simulink model "Baxter_brake_flex_sim"  (R2017b)
settings: Solver=ode8  StartTime=0.0  StopTime=T  FixedStep=0.0001  RelTol=5e-2  EnableMultiTasking=on
values from neighbouring files (symbols this model uses):
  A0 = zeros(6,1)    [friction_braking_analysis.m]    (also in friction_braking_analysis_flex.m)
  Ic = [(0.5*m*(3*r^2 + ht^2)) 0 0; 0 (0.5*m*(3*r^2 + ht^2)) 0;      0 0 0.5*m*r^2]    [friction_braking_analysis.m]    (also in friction_braking_analysis_flex.m; trap_traj_gen_check.m)
  Mc_inv = inv(Mc)    [friction_braking_analysis.m]    (also in friction_braking_analysis_flex.m; trap_traj_gen_check.m)
  N = length(lambda)-1    [trap_traj_gen_check.m]
  qdotIC = qIC    [friction_braking_analysis.m]    (also in friction_braking_analysis_flex.m)
  qIC = zeros(7,1)    [friction_braking_analysis.m]    (also in friction_braking_analysis_flex.m)
  qmdotIC = KN_inv*(Mdot*qddotIC + MassInertia*qjerkIC + Cdot*qdotIC +      C*qddotIC + Fdot + Ks*Ns*Ns*qdotIC + Jdot'*f + J'*fdot)    [friction_braking_analysis_flex.m]
  qmIC = KN_inv*(MassInertia*qddotIC + Cq + F + Ks*Ns*Ns*qIC +J'*f)    [friction_braking_analysis_flex.m]
  ric_tip = PTs    [friction_braking_analysis.m]    (also in friction_braking_analysis_flex.m; trap_traj_gen_check.m)
  Tb = 10*ones(7,1)    [friction_braking_analysis.m]    (also in friction_braking_analysis_flex.m)
  Tc = [1;1;1;1;0.5;0.5;0.5]    [friction_braking_analysis.m]    (also in friction_braking_analysis_flex.m)
  V0 = zeros(6,1)    [friction_braking_analysis.m]    (also in friction_braking_analysis_flex.m)
undefined symbols (not defined in the file or in its folder): qdotlimit, robot_const
libraries: simulink x1
settings Model: Creator=davidcarabis  LastModifiedBy=davidcarabis
settings SolverCC: MaxConsecutiveMinStep=10  ZeroCrossControl=EnableAll
settings DataIOCC: LimitDataPoints=on  SaveFormat=Array
settings OptimizationCC: LifeSpan=inf
settings DebuggingCC: ReadBeforeWriteMsg=DisableAll  WriteAfterWriteMsg=DisableAll  WriteAfterReadMsg=DisableAll  MultiTaskDSMMsg=none  SFUnexpectedBacktrackingDiag=warning  SFNoUnconditionalDefaultTransitionDiag=warning  SFExecutionAtInitializationDiag=none
settings HardwareCC: ProdBitPerPointer=32  ProdBitPerSizeT=32  ProdBitPerPtrDiffT=32  ProdLargestAtomicFloat=None  ProdIntDivRoundTo=Undefined  ProdEndianess=Unspecified  ProdWordSize=32  ProdHWDeviceType=32-bit Generic
settings ModelReferenceCC: UpdateModelReferenceTargets=IfOutOfDate  PropagateSignalLabelsOutOfModel=off
settings SFSimCC: SFSimEcho=off
settings CodeAppCC: StateflowObjectComments=on
settings GRTTargetCC: TargetLangStandard=C89/C90 (ANSI)  GeneratePreprocessorConditionals=Disable all
settings ConfigComp: CovMetricSettings=dw  CovHtmlReporting=on  CovSaveCumulativeToWorkspaceVar=on  CovSaveSingleToWorkspaceVar=on  CovExternalEMLEnable=off

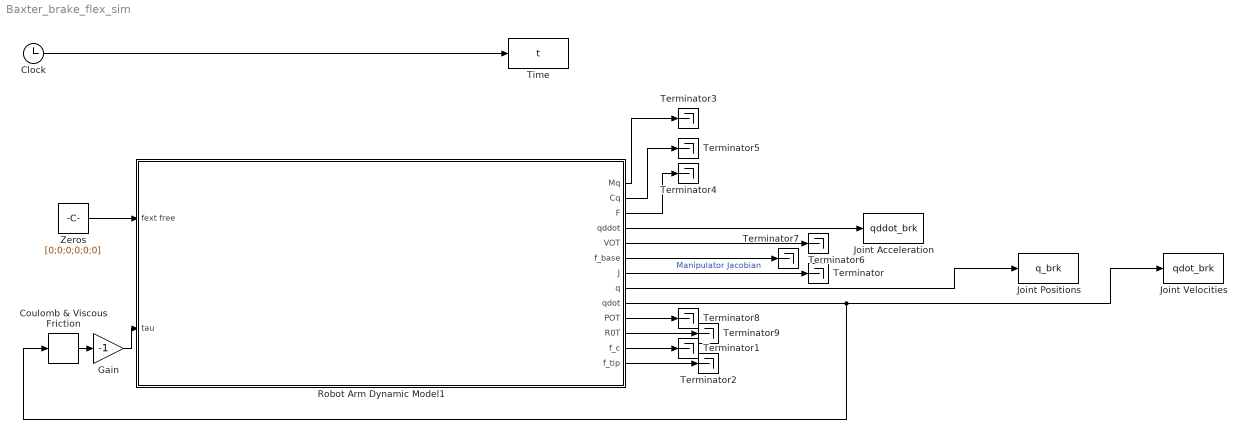
== system Baxter_brake_flex_sim ==
  Clock : Clock
  Coulomb & Viscous Friction : simulink/Discontinuities/Coulomb & Viscous Friction  offset=[Tc(1) Tc(2) Tc(3) Tc(4) Tc(5) Tc(6) Tc(7)]  gain=[Tb(1) Tb(2) Tb(3) Tb(4) Tb(5) Tb(6) Tb(7)]
      settings: SourceProductName=Simulink
  Gain : Gain  Gain=-1
  Joint Acceleration : ToWorkspace  VariableName=qddot_brk  SampleTime=-1
  Joint Positions : ToWorkspace  VariableName=q_brk  SampleTime=-1
  Joint Velocities : ToWorkspace  VariableName=qdot_brk  SampleTime=-1
  Robot Arm Dynamic Model1 : Subsystem
  Terminator{,1..9} (10 alike) : Terminator
  Time : ToWorkspace  VariableName=t  SampleTime=-1
  Zeros : Constant  Value=[0;0;0;0;0;0]
  wires:
  Clock/1 -> Time/1
  Robot Arm Dynamic Model1/9(qdot) -> Coulomb & Viscous Friction/1, Joint Velocities/1
  Robot Arm Dynamic Model1/8(q) -> Joint Positions/1
  Zeros/1 -> Robot Arm Dynamic Model1/1(fext free)
  Robot Arm Dynamic Model1/4(qddot) -> Joint Acceleration/1
  Robot Arm Dynamic Model1/7(J) -> Terminator/1  "Manipulator Jacobian"
  Robot Arm Dynamic Model1/12(f_c) -> Terminator1/1
  Robot Arm Dynamic Model1/13(f_tip) -> Terminator2/1
  Robot Arm Dynamic Model1/1(Mq) -> Terminator3/1
  Robot Arm Dynamic Model1/2(Cq) -> Terminator5/1
  Robot Arm Dynamic Model1/3(F) -> Terminator4/1
  Robot Arm Dynamic Model1/5(VOT) -> Terminator6/1
  Robot Arm Dynamic Model1/6(f_base) -> Terminator7/1
  Robot Arm Dynamic Model1/10(POT) -> Terminator8/1
  Robot Arm Dynamic Model1/11(R0T) -> Terminator9/1
  Coulomb & Viscous Friction/1 -> Gain/1
  Gain/1 -> Robot Arm Dynamic Model1/2(tau)

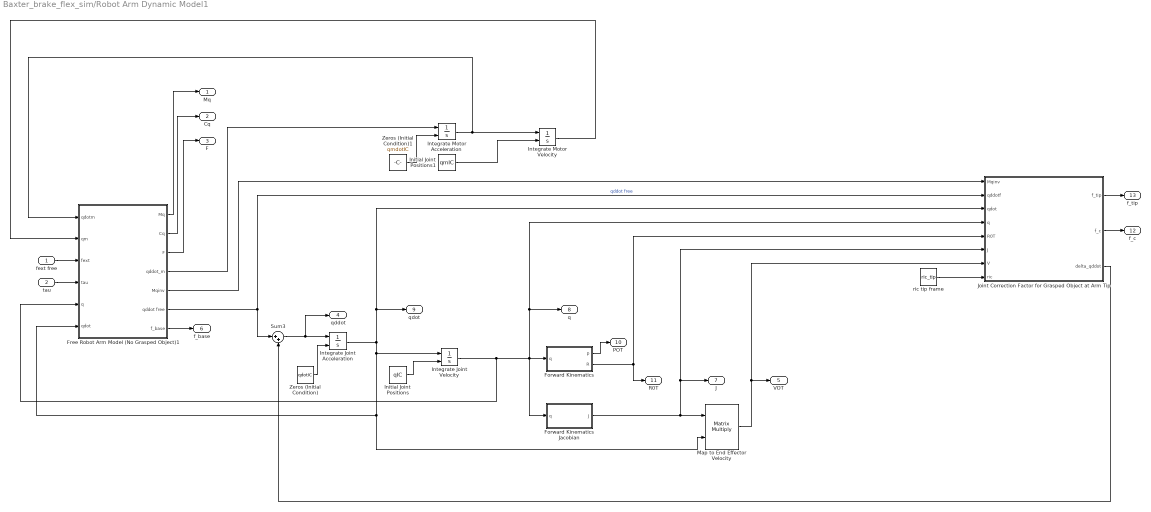
== system Baxter_brake_flex_sim/Robot Arm Dynamic Model1 ==
  fext free : Inport
  tau : Inport  Port=2
  Forward Kinematics : Subsystem  mask{H=robot_const.kin.H, P=robot_const.kin.P}
      mask prompts: H "Actuator Axes"; P "Actuator Displacements"
  Forward Kinematics Jacobian : Subsystem  mask{H=robot_const.kin.H, P=robot_const.kin.P}
      mask prompts: H "Actuator Axes"; P "Actuator Displacements"
  Free Robot Arm Model (No Grasped Object)1 : Subsystem
  Initial Joint Positions : Constant  Value=qIC
  Initial Joint Positions1 : Constant  Value=qmIC
  Integrate Joint Acceleration : Integrator  InitialConditionSource=external  InitialCondition=[0;0;0;0;0;0;0]
  Integrate Joint Velocity : Integrator  InitialConditionSource=external  InitialCondition=[0;0;0;0;0;0;0]
  Integrate Motor Acceleration : Integrator  InitialConditionSource=external  InitialCondition=[0;0;0;0;0;0;0]  UpperSaturationLimit=qdotlimit(:,2).*N  LowerSaturationLimit=qdotlimit(:,1).*N
  Integrate Motor Velocity : Integrator  InitialConditionSource=external  InitialCondition=[0;0;0;0;0;0;0]
  Joint Correction Factor for Grasped Object at Arm Tip : Subsystem  mask{Ic=Ic, Mcinv=Mc_inv}
  Map to End Effector Velocity : Product  Multiplication=Matrix(*)
  Sum3 : Sum  Inputs=|++
  Zeros (Initial Condition) : Constant  Value=qdotIC
  Zeros (Initial Condition)1 : Constant  Value=qmdotIC
  ric tip frame : Constant  Value=ric_tip
  Mq : Outport
  Cq : Outport  Port=2
  F : Outport  Port=3
  qddot : Outport  Port=4
  VOT : Outport  Port=5
  f_base : Outport  Port=6
  J : Outport  Port=7
  q : Outport  Port=8
  qdot : Outport  Port=9
  POT : Outport  Port=10
  R0T : Outport  Port=11
  f_c : Outport  Port=12
  f_tip : Outport  Port=13
  wires:
  Forward Kinematics/1(p) -> POT/1
  Integrate Joint Velocity/1 -> Free Robot Arm Model (No Grasped Object)1/5("q "), Forward Kinematics Jacobian/1(q), Forward Kinematics/1(q), Joint Correction Factor for Grasped Object at Arm Tip/4(q), q/1
  Zeros (Initial Condition)/1 -> Integrate Joint Acceleration/2
  fext free/1 -> Free Robot Arm Model (No Grasped Object)1/3(fext)
  Initial Joint Positions/1 -> Integrate Joint Velocity/2
  Forward Kinematics Jacobian/1(J) -> J/1, Joint Correction Factor for Grasped Object at Arm Tip/6(J), Map to End Effector Velocity/1
  Map to End Effector Velocity/1 -> Joint Correction Factor for Grasped Object at Arm Tip/7(V), VOT/1
  Integrate Joint Acceleration/1 -> Free Robot Arm Model (No Grasped Object)1/6(qdot), Map to End Effector Velocity/2, Integrate Joint Velocity/1, Joint Correction Factor for Grasped Object at Arm Tip/3(qdot), qdot/1
  tau/1 -> Free Robot Arm Model (No Grasped Object)1/4(tau)
  Forward Kinematics/2(R) -> Joint Correction Factor for Grasped Object at Arm Tip/5(R0T), R0T/1
  Free Robot Arm Model (No Grasped Object)1/7(f_base) -> f_base/1
  Free Robot Arm Model (No Grasped Object)1/5(Mqinv) -> Joint Correction Factor for Grasped Object at Arm Tip/1(Mqinv)
  Free Robot Arm Model (No Grasped Object)1/1(Mq) -> Mq/1
  Free Robot Arm Model (No Grasped Object)1/2(Cq) -> Cq/1
  Free Robot Arm Model (No Grasped Object)1/3(F) -> F/1
  Free Robot Arm Model (No Grasped Object)1/6(qddot free) -> Joint Correction Factor for Grasped Object at Arm Tip/2(qddotf), Sum3/1  "qddot free"
  Sum3/1 -> qddot/1, Integrate Joint Acceleration/1
  Joint Correction Factor for Grasped Object at Arm Tip/3(delta_qddot) -> Sum3/2
  Joint Correction Factor for Grasped Object at Arm Tip/2(f_c) -> f_c/1
  Joint Correction Factor for Grasped Object at Arm Tip/1(f_tip) -> f_tip/1
  ric tip frame/1 -> Joint Correction Factor for Grasped Object at Arm Tip/8(ric)
  Integrate Motor Acceleration/1 -> Free Robot Arm Model (No Grasped Object)1/1(qdotm), Integrate Motor Velocity/1
  Integrate Motor Velocity/1 -> Free Robot Arm Model (No Grasped Object)1/2(qm)
  Initial Joint Positions1/1 -> Integrate Motor Velocity/2
  Free Robot Arm Model (No Grasped Object)1/4(qddot_m) -> Integrate Motor Acceleration/1
  Zeros (Initial Condition)1/1 -> Integrate Motor Acceleration/2

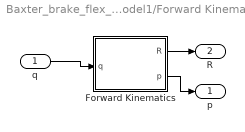
== system Baxter_brake_flex_sim/Robot Arm Dynamic Model1/Forward Kinematics ==
  q : Inport
  Forward Kinematics : MATLAB Function  TreatAsAtomicUnit=on
  p : Outport
  R : Outport  Port=2
  wires:
  q/1 -> Forward Kinematics/1(q)
  Forward Kinematics/2(p) -> p/1
  Forward Kinematics/1(R) -> R/1

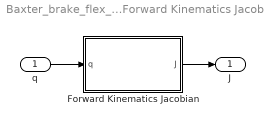
== system Baxter_brake_flex_sim/Robot Arm Dynamic Model1/Forward Kinematics Jacobian ==
  q : Inport
  Forward Kinematics Jacobian : MATLAB Function  TreatAsAtomicUnit=on
  J : Outport
  wires:
  q/1 -> Forward Kinematics Jacobian/1(q)
  Forward Kinematics Jacobian/1(J) -> J/1

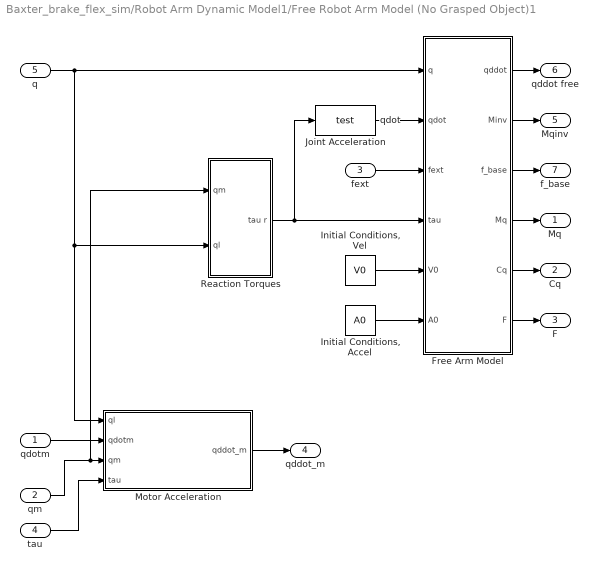
== system Baxter_brake_flex_sim/Robot Arm Dynamic Model1/Free Robot Arm Model (No Grasped Object)1 ==
  qdotm : Inport
  qm : Inport  Port=2
  fext : Inport  Port=3
  tau : Inport  Port=4
  "q " : Inport  Port=5
  qdot : Inport  Port=6
  Free Arm Model : Subsystem  mask{h=robot_const.kin.H, p=robot_const.kin.P, m=robot_const.mprops.m, c=robot_const.mprops.c, I=robot_const.mprops.I, Im=robot_const.mprops.Im, N=robot_const.mprops.N}
      mask prompts: h "Actuator Axes"; p "Actuator Displacements"; m "Link Masses"; c "Link COM"; I "Link Inertia"; N "Gear Ratio"
  "Initial Conditions, Accel" : Constant  Value=A0
  "Initial Conditions, Vel" : Constant  Value=V0
  Joint Acceleration : ToWorkspace  VariableName=test  SampleTime=-1
  Motor Acceleration : Subsystem  mask{Im=robot_const.mprops.Im, N=robot_const.mprops.N, K=robot_const.mprops.K}
      mask prompts: Im "Motor Inertias"; N "Gear Ratios"; K "Joint Stiffnesses"
  Reaction Torques : Subsystem  mask{N=robot_const.mprops.N, K=robot_const.mprops.K}
      mask prompts: N "Gear Ratios"; K "Joint Stiffnesses"
  Mq : Outport
  Cq : Outport  Port=2
  F : Outport  Port=3
  qddot_m : Outport  Port=4
  Mqinv : Outport  Port=5
  qddot free : Outport  Port=6
  f_base : Outport  Port=7
  wires:
  "q "/1 -> Reaction Torques/2(ql), Motor Acceleration/1(ql), Free Arm Model/1(q)
  fext/1 -> Free Arm Model/3(fext)
  qdot/1 -> Free Arm Model/2(qdot)
  "Initial Conditions, Vel"/1 -> Free Arm Model/5(V0)
  "Initial Conditions, Accel"/1 -> Free Arm Model/6(A0)
  Free Arm Model/1(qddot) -> qddot free/1
  Free Arm Model/2(Minv) -> Mqinv/1
  Free Arm Model/3(f_base) -> f_base/1
  Free Arm Model/4(Mq) -> Mq/1
  Free Arm Model/5(Cq) -> Cq/1
  Free Arm Model/6(F) -> F/1
  tau/1 -> Motor Acceleration/4(tau)
  Motor Acceleration/1(qddot_m) -> qddot_m/1
  qm/1 -> Reaction Torques/1(qm), Motor Acceleration/3(qm)
  qdotm/1 -> Motor Acceleration/2(qdotm)
  Reaction Torques/1(tau r) -> Joint Acceleration/1, Free Arm Model/4(tau)

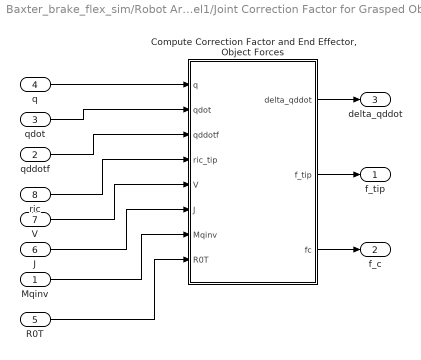
== system Baxter_brake_flex_sim/Robot Arm Dynamic Model1/Joint Correction Factor for Grasped Object at Arm Tip ==
  Mqinv : Inport
  qddotf : Inport  Port=2
  qdot : Inport  Port=3
  q : Inport  Port=4
  R0T : Inport  Port=5
  J : Inport  Port=6
  V : Inport  Port=7
  ric : Inport  Port=8
  "Compute Correction Factor and End Effector, Object Forces" : MATLAB Function  TreatAsAtomicUnit=on
  f_tip : Outport
  f_c : Outport  Port=2
  delta_qddot : Outport  Port=3
  wires:
  q/1 -> "Compute Correction Factor and End Effector, Object Forces"/1(q)
  "Compute Correction Factor and End Effector, Object Forces"/1(delta_qddot) -> delta_qddot/1
  J/1 -> "Compute Correction Factor and End Effector, Object Forces"/6(J)
  qddotf/1 -> "Compute Correction Factor and End Effector, Object Forces"/3(qddotf)
  ric/1 -> "Compute Correction Factor and End Effector, Object Forces"/4(ric_tip)
  qdot/1 -> "Compute Correction Factor and End Effector, Object Forces"/2(qdot)
  V/1 -> "Compute Correction Factor and End Effector, Object Forces"/5(V)
  Mqinv/1 -> "Compute Correction Factor and End Effector, Object Forces"/7(Mqinv)
  R0T/1 -> "Compute Correction Factor and End Effector, Object Forces"/8(R0T)
  "Compute Correction Factor and End Effector, Object Forces"/2(f_tip) -> f_tip/1
  "Compute Correction Factor and End Effector, Object Forces"/3(fc) -> f_c/1

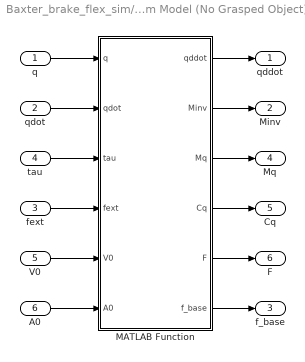
== system Baxter_brake_flex_sim/Robot Arm Dynamic Model1/Free Robot Arm Model (No Grasped Object)1/Free Arm Model ==
  q : Inport
  qdot : Inport  Port=2
  fext : Inport  Port=3
  tau : Inport  Port=4
  V0 : Inport  Port=5
  A0 : Inport  Port=6
  MATLAB Function : MATLAB Function  TreatAsAtomicUnit=on
  qddot : Outport
  Minv : Outport  Port=2
  f_base : Outport  Port=3
  Mq : Outport  Port=4
  Cq : Outport  Port=5
  F : Outport  Port=6
  wires:
  MATLAB Function/1(qddot) -> qddot/1
  q/1 -> MATLAB Function/1(q)
  fext/1 -> MATLAB Function/4(fext)
  tau/1 -> MATLAB Function/3(tau)
  V0/1 -> MATLAB Function/5(V0)
  qdot/1 -> MATLAB Function/2(qdot)
  A0/1 -> MATLAB Function/6(A0)
  MATLAB Function/2(Minv) -> Minv/1
  MATLAB Function/6(f_base) -> f_base/1
  MATLAB Function/3(Mq) -> Mq/1
  MATLAB Function/4(Cq) -> Cq/1
  MATLAB Function/5(F) -> F/1

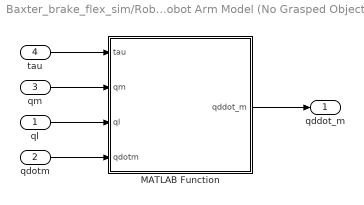
== system Baxter_brake_flex_sim/Robot Arm Dynamic Model1/Free Robot Arm Model (No Grasped Object)1/Motor Acceleration ==
  ql : Inport
  qdotm : Inport  Port=2
  qm : Inport  Port=3
  tau : Inport  Port=4
  MATLAB Function : MATLAB Function  TreatAsAtomicUnit=on
  qddot_m : Outport
  wires:
  ql/1 -> MATLAB Function/3(ql)
  tau/1 -> MATLAB Function/1(tau)
  qm/1 -> MATLAB Function/2(qm)
  MATLAB Function/1(qddot_m) -> qddot_m/1
  qdotm/1 -> MATLAB Function/4(qdotm)

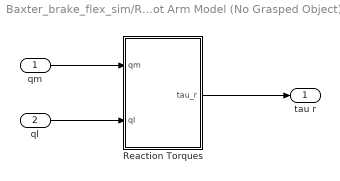
== system Baxter_brake_flex_sim/Robot Arm Dynamic Model1/Free Robot Arm Model (No Grasped Object)1/Reaction Torques ==
  qm : Inport
  ql : Inport  Port=2
  Reaction Torques : MATLAB Function  TreatAsAtomicUnit=on
  tau r : Outport
  wires:
  qm/1 -> Reaction Torques/1(qm)
  ql/1 -> Reaction Torques/2(ql)
  Reaction Torques/1(tau_r) -> tau r/1

== matlab function Baxter_brake_flex_sim/Robot Arm Dynamic Model1/Forward Kinematics/Forward Kinematics ==
  data: R output; q input; p output; H parameter; P parameter
function [R, p] = FwdKin(q,H,P)
%#codegen

% Generates robot pose from forward Kinematics
% Inputs:
% q: vector of joint positions
% H: matrix of joint unit vectors
% P: matrix of joint offsets
%
% Outputs:
% R: orientation (rotation matrix)
% P: position
%
%%%%%%%%%%%%%%%%%%%%%%%%%%%%%%%%%%%%%%%%%%%%%%%%%%%%%%%%%%%%%%%%%%%%%%%%%%%

    n = size(H,2);
    
    p = P(:,1);
    R = eye(3);
        
    for i=1:n
        R = R*rot(H(:,i),q(i));
        p = p + R*P(:,i+1);
    end
    
end

== matlab function Baxter_brake_flex_sim/Robot Arm Dynamic Model1/Forward Kinematics Jacobian/Forward Kinematics Jacobian ==
  data: J output; q input; H parameter; P parameter
function J = robotjacobian(q,H,P)
%#codegen

% Generates manipulator Jacobian using forward kinematics.
%
% Inputs: 
% q: vector of joint positions
% H: matrix of joint unit vectors
% P: matrix of joint offsets
%
% Outputs:
% J: manipulator Jacobian

%%%%%%%%%%%%%%%%%%%%%%%%%%%%%%%%%%%%%%%%%%%%%%%%%%%%%%%%%%%%%%%%%%%%%%%%%%%
    n = size(H,2);
    
    p = P(:,1);
    R = eye(3);
    
    hi = zeros(3,n);
    pOi = P;
        
    for i=1:n
        R = R*rot(H(:,i),q(i));
        p = p + R*P(:,i+1);
        pOi(:,i+1) = p;
        hi(:,i) = R*H(:,i);
    end
    
    pOT = pOi(:,end);
    J = zeros(6,n);
    
    for i=1:n
        J(:,i) = [hi(:,i); hat(hi(:,i))*(pOT - pOi(:,i))];
    end
    
end

== matlab function Baxter_brake_flex_sim/Robot Arm Dynamic Model1/Free Robot Arm Model (No Grasped Object)1/Free Arm Model/MATLAB Function ==
  data: q input; qddot output; qdot input; tau input; fext input; h parameter; p parameter; V0 input; A0 input; I parameter; m parameter; c parameter; Minv output; Mq output; Cq output; F output; f_base output; Im parameter; N parameter
function [qddot,Minv,Mq,Cq,F,f_base] = fcn(q,qdot,tau,fext,h,p,V0,A0,I,m,c,Im,N)
%#codegen

% This code computes the free dynamics of the Baxter arm using the N-E
% formulation. The free dynamics assumption is that there is no load at the
% tip of the manipulator arm.
%
% The N-E formulation is as follows for the ith joint:
% f_i = P_i*A_i + B_i
% First, a forward sweep computes spatial velocity of each point. 
% Next, a reverse sweep computes P, B for each joint.
% Finally, a forward sweep computes spatial acceleration, force, and joint
% acceleration.
%
% Inputs: 
% q: joint positions
% qdot: joint velocities
% tau: applied joint torques from motor/controller
% fext: external spatial force (should be set to zero)
% h: joint vectors of rotation
% p: joint offsets
% V0: spatial velocity initial condition
% A0: spatial acceleration initial condition
% I: equivalent manipulator link inertia matrices (accounts for motor 
%       inertia), at center of mass, represented in the ith frame for the
%       ith link
% m: manpulator link masses
% c: vectors from ith frame to ith link center of mass, represented in ith
%       frame
%
% Outputs:
% qddot: joint accelerations for free manipulator arm model
% Minv: inverse of the manipulator arm mass inertia matrix - this is needed
%       for the joint acceleration correction due to load at the tip
% f_base: spatial force at arm base

%%%%%%%%%%%%%%%%%%%%%%%%%%%%%%%%%%%%%%%%%%%%%%%%%%%%%%%%%%%%%%%%%%%%%%%%%%%

% Generate H, PHI block matrices

H1 = [h(:,1); 0;0;0]; H2 = [h(:,2); 0;0;0]; H3 = [h(:,3); 0;0;0]; 
H4 = [h(:,4); 0;0;0]; H5 = [h(:,5); 0;0;0]; H6 = [h(:,6); 0;0;0]; 
H7 = [h(:,7); 0;0;0];

H = [H1 zeros(6,6); zeros(6,1) H2 zeros(6,5); zeros(6,2) H3 zeros(6,4); ...
    zeros(6,3) H4 zeros(6,3); zeros(6,4) H5 zeros(6,2); zeros(6,5) H6 ...
    zeros(6,1); zeros(6,6) H7];

PHI = phi_gen(q,h,p);

N = diag(N);

%% Forward Sweep - Compute V,a,b, M
% V is spatial velocity of each joint.
% a,b are terms that will be used in later computations.
% Compute mass-inertia matrices for each link (M)

V = zeros(6,7);
Vtemp = V0;
Vprev = V0;
a = zeros(6,7);
b = zeros(6,7);
M = zeros(6,6,7);
M_motors = zeros(6,6,7);

for k = 1:7
   PHI_TEMP = PHI((6*(k) - 5):(6*(k)),(6*(k) - 5):(6*(k)));
   Htemp = H((6*(k) - 5):(6*(k)),k);
   Vtemp = PHI_TEMP*Vtemp + Htemp*qdot(k);
   V(:,k) = Vtemp;
   
   R = rot(H(:,k),q(k));
   
   a(:,k) = [crossmat(R'*Vprev(1:3))*(Vtemp(1:3));...
        R'*crossmat(Vprev(1:3))*(crossmat(Vprev(1:3))*p(:,k))];
   Vprev = Vtemp;
   
   b(:,k) = [crossmat(Vtemp(1:3))*I(:,:,k)*Vtemp(1:3); ...
        m(k)*crossmat(Vtemp(1:3))*crossmat(Vtemp(1:3))*c(:,k)];
    
    
    M(:,:,k) =  [I(:,:,k) m(k)*crossmat(c(:,k)); ...
        -m(k)*crossmat(c(:,k)) m(k)*eye(3,3)];
    M_motors(:,:,k) = [(I(:,:,k)+Im(k)*N(k,k)^2*h(:,k)*h(:,k)') m(k)*crossmat(c(:,k)); ...
        -m(k)*crossmat(c(:,k)) m(k)*eye(3,3)];
end

%% Backward Sweep for P, B
% Find P, B for each joint using reverse sweep.

F = -friction_adjust_Baxter(zeros(7,1),N*qdot);

P = zeros(6,6,7);
B = zeros(6,6,7);

% Handle Boundary Condition First
PHIT7 = [eye(3,3) zeros(3,3); -eye(3,3)*crossmat(p(:,8)) eye(3,3)];
P(:,:,7) = M(:,:,7);
B(:,7) = PHIT7'*fext + b(:,7);

% reverse sweep to compute other terms
for k = 6:-1:1
    PHI_TEMP = PHI((6*(k) +1):(6*(k)+6),(6*(k) +1):(6*(k) + 6));
    Htemp = H((6*(k) +1):(6*(k))+6,k+1);
    P(:,:,k) = M(:,:,k) + PHI_TEMP'*P(:,:,k+1)*PHI_TEMP - ...
        (PHI_TEMP'*P(:,:,k+1)*Htemp*Htemp'*P(:,:,k+1)*PHI_TEMP)/...
        (Htemp'*P(:,:,k+1)*Htemp);
    
    B(:,k) = PHI_TEMP'*(P(:,:,k+1)*a(:,k+1) + B(:,k+1)) + b(:,k) + ...
        (PHI_TEMP'*P(:,:,k+1)*Htemp*(tau(k+1) - Htemp'*...
        (P(:,:,k+1)*a(:,k+1) + B(:,k+1))))/(Htemp'*P(:,:,k+1)*Htemp);
    
end

%% Sweep Forward for qddot, A, f
% qddot is joint acceleration
% A is spatial acceleration at each joint
% f is spatial force at each joint

qddot = zeros(7,1);
Atemp = A0;
atemp = zeros(6,1);
f = zeros(6,7);

for k = 1:7
    atemp = a(:,k);
    PHI_TEMP = PHI((6*(k) - 5):(6*(k)),(6*(k) - 5):(6*(k)));
    Htemp = H((6*(k) - 5):(6*(k)),k);
    qddot(k) = (tau(k) - Htemp'*P(:,:,k)*PHI_TEMP*Atemp - Htemp'*...
        (P(:,:,k)*atemp + B(:,k)))/(Htemp'*P(:,:,k)*Htemp);
    
    Atemp = PHI_TEMP*Atemp + Htemp*qddot(k) + a(:,k);
    f(:,k) = P(:,:,k)*Atemp + B(:,k);
end

% Transform to base frame:
f_base = [eye(3) crossmat(-p(:,1)); zeros(3) eye(3)]*f(:,1);

%% gemerate inverse of manpulator arm mass-inertia matrix
% This must be computed for finding the joint acceleration correction due
% to loading at the tip.

PHI = PHI(:,7:end);

M_NE = zeros(42,42);
% % Do Not account for motor inertias
% M_NE(1:6,1:6) = M(:,:,1); M_NE(7:12,7:12) = M(:,:,2); 
% M_NE(13:18,13:18) = M(:,:,3); M_NE(19:24,19:24) = M(:,:,4);
% M_NE(25:30,25:30) = M(:,:,5); M_NE(31:36,31:36) = M(:,:,6); 
% M_NE(37:42,37:42) = M(:,:,7);

% Account for Motor Inertias
M_NE(1:6,1:6) = M_motors(:,:,1); M_NE(7:12,7:12) = M_motors(:,:,2); 
M_NE(13:18,13:18) = M_motors(:,:,3); M_NE(19:24,19:24) = M_motors(:,:,4);
M_NE(25:30,25:30) = M_motors(:,:,5); M_NE(31:36,31:36) = M_motors(:,:,6); 
M_NE(37:42,37:42) = M_motors(:,:,7);

MassInertia = H'*PHI'*M_NE*PHI*H;
Mq = MassInertia;
Minv = inv(MassInertia);
Cq = H'*PHI'*(M_NE*PHI*a(:) + b(:));

== matlab function Baxter_brake_flex_sim/Robot Arm Dynamic Model1/Joint Correction Factor for Grasped Object at Arm Tip/Compute Correction Factor and End Effector, Object Forces ==
  data: q input; qdot input; qddotf input; ric_tip input; delta_qddot output; V input; Ic parameter; Mcinv parameter; J input; Mqinv input; R0T input; f_tip output; fc output
function [delta_qddot,f_tip,fc]  = fcn(q,qdot,qddotf,ric_tip,V,Ic,Mcinv,J,Mqinv,R0T)
%#codegen

% This code computes the joint accleration correction factor for the
% Baxter Arm dynamic model due to a rigidly grasped mass at the end
% effector. This correction can then be added to the free arm model joint
% acceleration.
%
% Outputs:
% delta_qddot: joint acceleration correction due to mass at tip
% f_tip: end effector spatial force applied to the environment
%       (torque,force)^T
% fc: spatial force experienced by mass at center frame C (torque,force)^T
%
% Inputs: 
% ric_tip: vector from contact point to center frame C of object,
%       represented in the tip (end effector) frame
% V: end effector spatial velocity (rad/s, m/s)^T
% Ic: inertia matrix of captured object represented in C frame
% Mcinv: inverse of the mass-inertia matrix of the captured object
% q: current joint positions
% qdot: current joint velocities 
% J: current robot manipulator Jacobian
% qddotf: current joint accelerations from free robot arm model
% Mqinv: inverse of the mass-inertia matrix of the robot arm
% R0T: rotation matrix representing orientation of end effector with
%       respect to origin frame
%%%%%%%%%%%%%%%%%%%%%%%%%%%%%%%%%%%%%%%%%%%%%%%%%%%%%%%%%%%%%%%%%%%%%%%%%%%

% Compute Jacobian transformation from object frame C to to arm tip frame
% (A) and the derivative (Adiff)
A = [[R0T zeros(3)];[R0T*hat(ric_tip) R0T]];

Adiff = baxter_Adiff(q,qdot,ric_tip);

% Propogate tip velocity to object frame C
Vc = A\V;

% Compute spatial force at object frame C due to centrifugal and Coriolis
% effects
bc = [[hat(Vc(1:3))*Ic*Vc(1:3)]; zeros(3,1)];

% Compute derivative of manipulator Jacobian
Jdot = baxter_Jdiff(q,qdot);

% Compute tip force, propogate to C frame, and compute correction factor
f_tip = inv(A*Mcinv*A' + J*Mqinv*J')*(J*qddotf + Jdot*qdot - Adiff*Vc+ A*Mcinv*bc);
fc = A'*f_tip;
delta_qddot = -Mqinv*J'*f_tip;

== matlab function Baxter_brake_flex_sim/Robot Arm Dynamic Model1/Free Robot Arm Model (No Grasped Object)1/Motor Acceleration/MATLAB Function ==
  data: tau input; qddot_m output; Im parameter; K parameter; N parameter; qm input; ql input; qdotm input
function qddot_m   = fcn(tau,Im,K,N,qm,ql,qdotm)
%#codegen

% This function computes the motor accelerations.
%
% Output: 
%   qddot_m: 7x1 vector of motor accelerations
%
% Input:
%   tau: 7x1 vector of input motor torques
%   Im: 7x1 vector of motor inertias
%   K: 7x1 vector of joint stiffnesses
%   N: 7x1 vector of gear ratios
%   qm: 7x1 vector of motor positions
%   ql: 7x1 vector of link positions

%%%%%%%%%%%%%%%%%%%%%%%%%%%%%%%%%%%%%%%%%%%%%%%%%%%%%%%%%%%%%%%%%%%%%%%%%%%

qddot_m = zeros(7,1);
tau_total = qddot_m;

Flink = friction_adjust_Baxter(zeros(7,1),qdotm);

tau = tau + Flink./N;

for n = 1:7
   qddot_m(n,1) = (tau(n) + K(n)*(N(n)*ql(n) - qm(n)))/Im(n); 
   tau_total(n,1) = (tau(n) + K(n)*(N(n)*ql(n) - qm(n)));
    
end

== matlab function Baxter_brake_flex_sim/Robot Arm Dynamic Model1/Free Robot Arm Model (No Grasped Object)1/Reaction Torques/Reaction Torques ==
  data: N parameter; tau_r output; K parameter; qm input; ql input
function tau_r = fcn(N,K,qm,ql)
%#codegen

% This block computes the reaction torque at each link using the gear
% ratios, joint stiffnesses (approximated as torsional springs), motor
% positions, and joint positions. 
%
% Outputs: 
% tau_r: 7x1 vector of reaction torques at links
%
% Inputs: 
% N: 7x1 vector of gear ratios
% K: 7x1 vector of joint stiffnesses
% qm: 7x1 vector of motor positions
% ql: 7x1 vector of joint positions

%%%%%%%%%%%%%%%%%%%%%%%%%%%%%%%%%%%%%%%%%%%%%%%%%%%%%%%%%%%%%%%%%%%%%%%%%%%
tau_r = zeros(7,1);
for n = 1:7
    tau_r(n,1) = N(n)*K(n)*(qm(n) - N(n)*ql(n));
end
